simulink model "ProgettoCompleto"  (R2022b)
settings: Solver=ode1  StartTime=0.0  StopTime=inf  FixedStep=0.001  RelTol=1e-9
PreLoadFcn:
  | params
InitFcn:
  | params
model workspace (MAT data in the model file):
  SL_ROS_VariableLengthArrays_MaxSizes.CommonInfo.ArrayTruncateAction = 'EmitWarning'
  SL_ROS_VariableLengthArrays_MaxSizes.MsgTypeMap = containers.Map
  SL_ROS_VariableLengthArrays_MaxSizes.MsgTypeMap.serialization.keys = {'sensor_msgs/CompressedImage'}
  SL_ROS_VariableLengthArrays_MaxSizes.MsgTypeMap.serialization.values{1}(1).PropertyName = 'Data'
  SL_ROS_VariableLengthArrays_MaxSizes.MsgTypeMap.serialization.values{1}(1).DataType = 'uint8'
  SL_ROS_VariableLengthArrays_MaxSizes.MsgTypeMap.serialization.values{1}(1).MaxLength = 300000
  SL_ROS_VariableLengthArrays_MaxSizes.MsgTypeMap.serialization.values{1}(2).PropertyName = 'Format'
  SL_ROS_VariableLengthArrays_MaxSizes.MsgTypeMap.serialization.values{1}(2).DataType = 'uint8'
  SL_ROS_VariableLengthArrays_MaxSizes.MsgTypeMap.serialization.values{1}(2).MaxLength = 128
  SL_ROS_VariableLengthArrays_MaxSizes.MsgTypeMap.serialization.uniformity = 0
  SL_ROS_VariableLengthArrays_MaxSizes.MsgTypeMap.serialization.keyType = 'char'
  SL_ROS_VariableLengthArrays_MaxSizes.MsgTypeMap.serialization.valueType = 'any'
undefined symbols (not defined in the file): gray, L, r, Rec, SDTV, sigbuilder_block, VelLeft, VelRight
libraries: robotlib x8, simulink_extras x8, dspstat3 x4, visiontextngfix x3, slpidlib x3, visiontransforms x2, visionconversions x2, dspmtrx3 x2, visionfilter x1, matrix_library x1, visionanalysis x1, visionstatistics x1
settings Model: Creator=domen  LastModifiedBy=gaetano
settings OptimizationCC: EnhancedBackFolding=on  PassReuseOutputArgsAs=Individual arguments  ZeroExternalMemoryAtStartup=off  ZeroInternalMemoryAtStartup=off  MaxStackSize=64  OptimizeBlockOrder=speed  DifferentSizesBufferReuse=on  OptimizationCustomize=off  EfficientTunableParamExpr=on
settings DebuggingCC: ParameterTunabilityLossMsg=error
settings HardwareCC: ProdBitPerPointer=32  ProdBitPerSizeT=32  ProdBitPerPtrDiffT=32  ProdLargestAtomicFloat=None  ProdIntDivRoundTo=Undefined  ProdEndianess=Unspecified  ProdWordSize=32  ProdHWDeviceType=Generic->Unspecified (assume 32-bit Generic)  UseEmbeddedCoderFeatures=off
settings RTWCC: Description=Embedded Coder  SystemTargetFile=ert.tlc  HardwareBoard=Robot Operating System (ROS)  TLCOptions="-aInlineSetEventsForThisBaseRateFcn=TLC_FALSE -aSuppressMultiTaskScheduler=TLC_FALSE  -aRateBasedStepFcn=0"  TemplateMakefile=ert_default_tmf  Toolchain=Catkin  TargetLang=C++
settings CodeAppCC: ForceParamTrailComments=on  IgnoreCustomStorageClasses=off  OperatorAnnotations=on  SimulinkDataObjDesc=on  SFDataObjDesc=on  InsertBlockDesc=on
settings ERTTargetCC: SupportNonInlinedSFcns=on

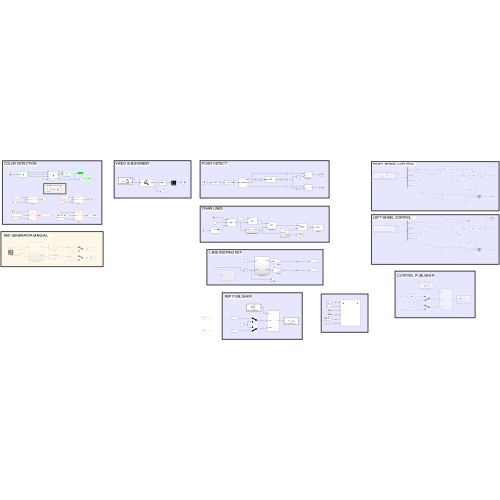
[thumbnail: Simulink's stored preview of the top-level diagram]
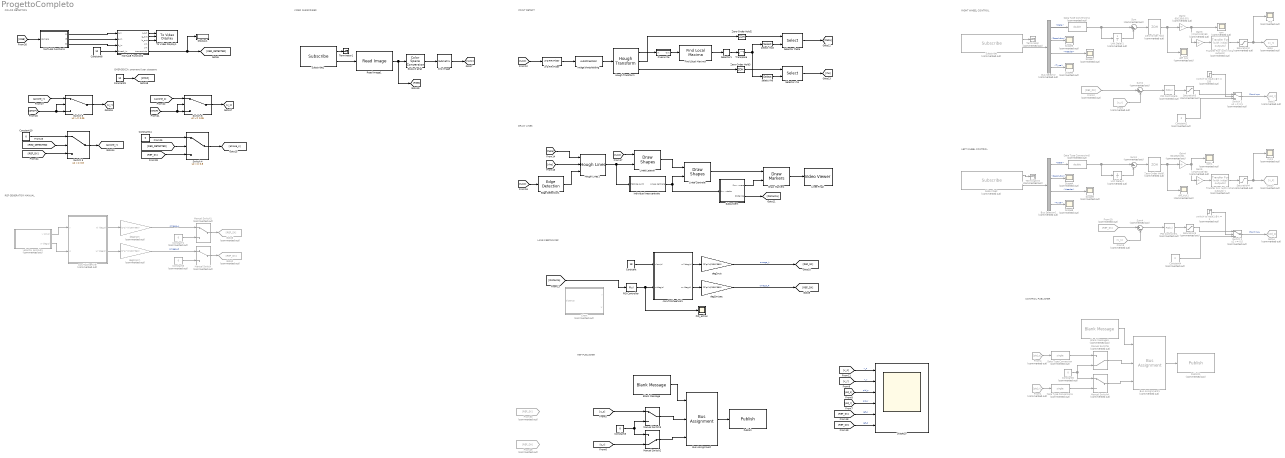
== system ProgettoCompleto ==
  note: VIDEO SUBSCRIBER
  note: POINT DETECT
  note: DRAW LINES
  note: LANE KEEPING REF
  note: REF PUBLISHER
  note: CONTROL PUBLISHER
  note: EMERGENZA: premere 0 per stoppare
  note: COLOR DETECTION
  note: REF GENERATOR MANUAL
  note: RIGHT WHEEL CONTROL
  note: LEFT WHEEL CONTROL
  2-D FIR Filter : visionfilter/2-D FIR Filter  separable=off  filtSrc=Specify via dialog  filterMtrx=[-1 0 1]  verticalFilter=[4 0]  horizontalFilter=[4 0]  outSize=Same as input port I  padType=Replicate  padSrc=Specify via dialog  padVal=0  method=Convolution  firstCoeffMode=Specify word length  firstCoeffWordLength=16  firstCoeffFracLength=14  firstCoeffSignedness=Signed  firstCoeffLastDataTypeStr=fixdt(1,16)  outputSignedness=Auto  accumLastDataTypeStr=Inherit: Same as product output  prodOutputMode=Binary point scaling  prodOutputWordLength=32  prodOutputFracLength=10  prodOutputLastDataTypeStr=fixdt([],32,10)  roundingMode=Floor  overflowMode=on  firstCoeffDataTypeStr=fixdt(1,16)  firstCoeffMin=[]  firstCoeffMax=[]  prodOutputDataTypeStr=fixdt([],32,10)  accumDataTypeStr=Inherit: Same as product output  outputMin=[]  outputMax=[]
  Blank Message : robotlib/Blank Message  messageClass=Message  entityType=duckietown_msgs/WheelsCmdStamped  messageType=duckietown_msgs/WheelsCmdStamped  SampleTime=-1  legacyBusStruct=off
      settings: LibrarySourceBlock=roslib/ROS/Blank Message
  Blank Message1 : robotlib/Blank Message  Commented=on  messageClass=Message  entityType=duckietown_msgs/WheelsCmdStamped  messageType=duckietown_msgs/WheelsCmdStamped  SampleTime=-1  legacyBusStruct=off
      settings: LibrarySourceBlock=roslib/ROS/Blank Message
  Bus Assignment : BusAssignment  AssignedSignals=VelLeft,VelRight
  Bus Assignment1 : BusAssignment  Commented=on  AssignedSignals=VelLeft,VelRight
  Bus Selector : BusSelector  Commented=on  OutputSignals=Data,Resolution,Header,Type
  Bus Selector1 : BusSelector  Commented=on  OutputSignals=Data,Resolution,Header,Type
  Chart : Stateflow chart  Commented=on  TreatAsAtomicUnit=on
  Clip image : matrix_library/Submatrix  RowSpan=Range of rows  RowStartMode=Offset from middle  RowStartIndex=15  RowEndMode=Last  RowEndIndex=1  ColSpan=All columns  ColStartMode=First  ColStartIndex=1  ColEndMode=Last  ColEndIndex=1
  Constant : Constant  Value=18
  Constant{1..2,4..5} (4 alike) : Constant  Commented=on  Value=0
  Constant10 : Constant  Value=0
  Constant11 : Constant  Value=0
  Constant3 : Constant  Value=0  OutDataTypeStr=single
  Constant6 : Constant  Commented=on  Value=0  OutDataTypeStr=single
  Constant8 : Constant  Value=10
  Constant9 : Constant  Value=10
  Data Type Conversion : DataTypeConversion  Commented=on  OutDataTypeStr=single  SaturateOnIntegerOverflow=off  RndMeth=Floor
  Data Type Conversion1 : DataTypeConversion  Commented=on  OutDataTypeStr=single  SaturateOnIntegerOverflow=off  RndMeth=Floor
  Data Type Conversion4 : DataTypeConversion  Commented=on  OutDataTypeStr=double  SaturateOnIntegerOverflow=off  RndMeth=Floor
  Data Type Conversion5 : DataTypeConversion  Commented=on  OutDataTypeStr=double  SaturateOnIntegerOverflow=off  RndMeth=Floor
  Display1 : Display
  Draw Markers : visiontextngfix/Draw Markers  shape=X-mark  size=3  fill=off  fillClrSource=Specify via dialog  display=White  intensity=200  color=[250 0 0]  opacity=0.6  viewport=Entire image  antialiasing=off  inType=Obsolete  imagePorts=One multidimensional signal  roundingMode=Floor  overflowMode=off  memoryMode=Specify word length  memoryWordLength=16  memoryFracLength=15  prodOutputMode=Binary point scaling  prodOutputWordLength=32  prodOutputFracLength=14
  Edge Detection1 : visionanalysis/Edge Detection  method=Sobel  outputType=Binary image  userDefinedThreshold=off  thresholdSource=Input port  threshold=20  thresholdTuning=4  edgeThinning=off  threshold_canny=[0.25 0.60]  autoPercent=70  sigma=1  roundingMode=Floor  overflowMode=off  prodOutputMode=Binary point scaling  prodOutputWordLength=32  prodOutputFracLength=8
  Find Local Maxima : visionstatistics/Find Local Maxima  num_peaks=2  nhood_size=[301 81]  src_thresh=Obsolete9b  src_thresh_inuse=Specify via dialog  threshold=1  inputIsHough=on  dt_peak=uint16  isOutVarDim=on  dt_count=uint16
  From : From  Commented=on  GotoTag=v_r
  From1 : From  Commented=on  GotoTag=pid_r
  From10 : From  Commented=on  GotoTag=REF_SX
  From2 : From  Commented=on  GotoTag=REF_DX
  From29 : From  Commented=on  GotoTag=REF_DX
  From3 : From  Commented=on  GotoTag=v_s
  From30 : From  Commented=on  GotoTag=REF_SX
  From4 : From  Commented=on  GotoTag=pid_s
  Gain2 : Gain  Commented=on  Gain=60/135/0.001
  Gain3 : Gain  Commented=on  Gain=(2*pi*0.03)/60
  Gain4 : Gain  Commented=on  Gain=60/135/0.001
  Gain5 : Gain  Commented=on  Gain=(2*pi*0.03)/60
  Goto : Goto  Commented=on  GotoTag=v_r
  Goto1 : Goto  Commented=on  GotoTag=pid_r
  Goto2 : Goto  Commented=on  GotoTag=REF_DX
  Goto3 : Goto  Commented=on  GotoTag=v_s
  Goto4 : Goto  Commented=on  GotoTag=pid_s
  Goto6 : Goto  Commented=on  GotoTag=REF_SX
  Hough Lines1 : visiontransforms/Hough Lines  sineCompMethod=Trigonometric function  thetaRes=pi/180  roundingMode=Nearest  overflowMode=on  firstCoeffMode=Specify word length  firstCoeffWordLength=16  prodOutputMode=Binary point scaling  prodOutputWordLength=32  prodOutputFracLength=16  firstCoeffFracLength=15
  Hough Transform : visiontransforms/Hough Transform  theta_res=pi/180  rho_res=1  out_theta_rho=on  outdtmode=single  roundingMode=Nearest  overflowMode=on  firstCoeffMode=Binary point scaling  firstCoeffWordLength=16  firstCoeffFracLength=14  secondCoeffMode=Binary point scaling  secondCoeffWordLength=32  secondCoeffFracLength=16  prodOutputMode=Binary point scaling  prodOutputWordLength=32  prodOutputFracLength=20  accumMode=Binary point scaling  accumWordLength=32  accumFracLength=20  outputMode=Binary point scaling  outputWordLength=16  outputFracLength=0  memoryMode=Binary point scaling  memoryWordLength=32  memoryFracLength=16
  Image thresholding : visionconversions/Autothreshold  operator=>  threshOut=off  effMetricOut=off  userDefinedRange=off  umin=50  umax=255  outOfRngOpt=Ignore  scaleThreshold=off  scaleFactor=1  roundingMode=Floor  overflowMode=off  P1Mode=Specify word length  P1WordLength=32  P1FracLength=30  P2Mode=Specify word length  P2WordLength=32  P2FracLength=22  P3Mode=Specify word length  P3WordLength=32  P3FracLength=14  P4Mode=Binary point scaling  P4WordLength=32  P4FracLength=15  Q1Mode=Specify word length  Q1WordLength=32  Q1FracLength=16  EMMode=Specify word length  EMWordLength=16  EMFracLength=14
  Individua linea centrale : Subsystem
  Linea Centrale : visiontextngfix/Draw Shapes  shape=Lines  fill=off  lineWidth=2  fillClrSource=Specify via dialog  display=White  intensity=200  color=[200 255 100]  opacity=0.6  viewport=Entire image  antialiasing=off  inType=Obsolete  imagePorts=One multidimensional signal  roundingMode=Floor  overflowMode=off  memoryMode=Specify word length  memoryWordLength=16  prodOutputMode=Binary point scaling  prodOutputWordLength=32  prodOutputFracLength=14  memoryFracLength=15
  Linee Finali : VideoViewer  colormapValue=gray(256)  FigPos=[342 823 793 695]
  Linee Laterali : visiontextngfix/Draw Shapes  shape=Lines  fill=off  lineWidth=2  fillClrSource=Specify via dialog  display=White  intensity=200  color=[200 255 100]  opacity=0.6  viewport=Entire image  antialiasing=off  inType=Obsolete  imagePorts=One multidimensional signal  roundingMode=Floor  overflowMode=off  memoryMode=Specify word length  memoryWordLength=16  prodOutputMode=Binary point scaling  prodOutputWordLength=32  prodOutputFracLength=14  memoryFracLength=15
  MATLAB Function1 : MATLAB Function  TreatAsAtomicUnit=on
  MATLAB Function2 : MATLAB Function  TreatAsAtomicUnit=on
  Manual Switch : ManualSwitch  Commented=on
  Manual Switch1 : ManualSwitch  Commented=on
  Manual Switch2 : ManualSwitch  CurrentSetting=0
  Manual Switch3 : ManualSwitch
  Manual Switch4 : ManualSwitch  Commented=on
  Manual Switch5 : ManualSwitch  Commented=on  CurrentSetting=0
  Overwrite : Subsystem
  PID Controller : slpidlib/PID Controller  Controller=P  Form=Parallel  TimeDomain=Continuous-time  UseExternalTs=off  SampleTime=-1  IntegratorMethod=Forward Euler  FilterMethod=Forward Euler  ControllerParametersSource=internal  P=0.70  I=1  UseKiTs=off  D=0.10  N=100  UseFilter=on  TunerSelectOption=Transfer Function Based (PID Tuner App)  InitialConditionSource=internal  InitialConditionForIntegrator=0  InitialConditionForFilter=0  DifferentiatorICPrevScaledInput=0  ExternalReset=none  TrackingMode=off  Kt=1  LimitOutput=off  SatLimitsSource=internal  UpperSaturationLimit=40  LowerSaturationLimit=-40  LinearizeAsGain=off  AntiWindupMode=none  Kb=1  LimitIntegrator=off  UpperIntegratorSaturationLimit=inf  LowerIntegratorSaturationLimit=-inf  PGainOutDataTypeStr=double  PProdOutDataTypeStr=double  POutMin=[]  POutMax=[]  IOutMin=[]  IOutMax=[]  DOutMin=[]  DOutMax=[]  NOutMin=[]  NOutMax=[]  SumOutMin=[]  SumOutMax=[]  SaturationOutMin=[]  SaturationOutMax=[]  PParamMin=[]  PParamMax=[]  IParamMin=[]  IParamMax=[]  DParamMin=[]  DParamMax=[]  NParamMin=[]  NParamMax=[]  KbParamMin=[]  KbParamMax=[]  KtParamMin=[]  KtParamMax=[]  KbOutMin=[]  KbOutMax=[]  KtOutMin=[]  KtOutMax=[]  IntegratorOutMin=[]  IntegratorOutMax=[]  FilterOutMin=[]  FilterOutMax=[]  SumI1OutMin=[]  SumI1OutMax=[]  SumI2OutMin=[]  SumI2OutMax=[]  SumI3OutMin=[]  SumI3OutMax=[]  SumI4OutMin=[]  SumI4OutMax=[]  SumDOutMin=[]  SumDOutMax=[]  DifferentiatorOutMin=[]  DifferentiatorOutMax=[]  FilterDiffOutCoefMin=[]  FilterDiffOutCoefMax=[]  ReciprocalOutMin=[]  ReciprocalOutMax=[]  SumDenOutMin=[]  SumDenOutMax=[]  SumNumOutMin=[]  SumNumOutMax=[]  DivideOutMin=[]  DivideOutMax=[]  UdiffTsProdOutMin=[]  UdiffTsProdOutMax=[]  NTsProdOutMin=[]  NTsProdOutMax=[]  UintegralTsProdOutMin=[]  UintegralTsProdOutMax=[]  UngainTsProdOutMin=[]  UngainTsProdOutMax=[]  ClampingZeroOutDataTypeStr=Inherit: Inherit via back propagation  ClampingZeroOutMin=[]  ClampingZeroOutMax=[]  FilterDenConstantOutDataTypeStr=Inherit: Inherit via back propagation  FilterDenConstantOutMin=[]  FilterDenConstantOutMax=[]  PCopyOutDataTypeStr=Inherit: Inherit via back propagation  PCopyOutMin=[]  PCopyOutMax=[]  NCopyOutDataTypeStr=Inherit: Inherit via back propagation  NCopyOutMin=[]  NCopyOutMax=[]  IntegratorContinuousStateAttributes=''  IntegratorStateMustResolveToSignalObject=off  IntegratorRTWStateStorageClass=Auto  FilterContinuousStateAttributes=''  FilterStateMustResolveToSignalObject=off  FilterRTWStateStorageClass=Auto  ParallelPVariant=InternalParameters  IdealPVariant=Disabled  IVariant=Disabled  DVariant=Disabled  IntegratorVariant=Disabled  SatVariant=Disabled  AWVariant=Disabled  PCopyVariant=Disabled  TRVariant=Disabled  FdbkBlocksVariant=Forward  IdealPFdbkVariant=Disabled  SatFdbkVariant=Disabled  DerivativeFilterVariant=Disabled  NVariant=Disabled  NCopyVariant=Disabled_SignalSpec  FilterICVariant=Disabled  IntegratorICVariant=Disabled  ExternalResetVariant=Disabled  TRSumVariant=Passthrough  SumFdbkVariant=Disabled  SumVariant=Passthrough_P  TsampFilterVariant=InternalTs  TsampNgainVariant=Passthrough  TsampIntegralVariant=Disabled_SignalSpec  ExternalSaturationOutDataTypeStr=Inherit: Same as second input
  PID Controller1 : slpidlib/PID Controller  Commented=on  Controller=PID  Form=Parallel  TimeDomain=Continuous-time  UseExternalTs=off  SampleTime=-1  IntegratorMethod=Forward Euler  FilterMethod=Forward Euler  ControllerParametersSource=internal  P=1.9500021729767  I=2.64652436503106  UseKiTs=off  D=0.143645278367384  N=3.78681783159113  UseFilter=on  TunerSelectOption=Transfer Function Based (PID Tuner App)  InitialConditionSource=internal  InitialConditionForIntegrator=0  InitialConditionForFilter=0  DifferentiatorICPrevScaledInput=0  ExternalReset=none  TrackingMode=off  Kt=1  LimitOutput=off  SatLimitsSource=internal  UpperSaturationLimit=inf  LowerSaturationLimit=-inf  LinearizeAsGain=on  AntiWindupMode=none  Kb=1  LimitIntegrator=off  UpperIntegratorSaturationLimit=inf  LowerIntegratorSaturationLimit=-inf  POutMin=[]  POutMax=[]  IOutMin=[]  IOutMax=[]  DOutMin=[]  DOutMax=[]  NOutMin=[]  NOutMax=[]  SumOutMin=[]  SumOutMax=[]  SaturationOutMin=[]  SaturationOutMax=[]  PParamMin=[]  PParamMax=[]  IParamMin=[]  IParamMax=[]  DParamMin=[]  DParamMax=[]  NParamMin=[]  NParamMax=[]  KbParamMin=[]  KbParamMax=[]  KtParamMin=[]  KtParamMax=[]  KbOutMin=[]  KbOutMax=[]  KtOutMin=[]  KtOutMax=[]  IntegratorOutMin=[]  IntegratorOutMax=[]  FilterOutMin=[]  FilterOutMax=[]  SumI1OutMin=[]  SumI1OutMax=[]  SumI2OutMin=[]  SumI2OutMax=[]  SumI3OutMin=[]  SumI3OutMax=[]  SumI4OutMin=[]  SumI4OutMax=[]  SumDOutMin=[]  SumDOutMax=[]  DifferentiatorOutMin=[]  DifferentiatorOutMax=[]  FilterDiffOutCoefMin=[]  FilterDiffOutCoefMax=[]  ReciprocalOutMin=[]  ReciprocalOutMax=[]  SumDenOutMin=[]  SumDenOutMax=[]  SumNumOutMin=[]  SumNumOutMax=[]  DivideOutMin=[]  DivideOutMax=[]  UdiffTsProdOutMin=[]  UdiffTsProdOutMax=[]  NTsProdOutMin=[]  NTsProdOutMax=[]  UintegralTsProdOutMin=[]  UintegralTsProdOutMax=[]  UngainTsProdOutMin=[]  UngainTsProdOutMax=[]  ClampingZeroOutDataTypeStr=Inherit: Inherit via back propagation  ClampingZeroOutMin=[]  ClampingZeroOutMax=[]  FilterDenConstantOutDataTypeStr=Inherit: Inherit via back propagation  FilterDenConstantOutMin=[]  FilterDenConstantOutMax=[]  PCopyOutDataTypeStr=Inherit: Inherit via back propagation  PCopyOutMin=[]  PCopyOutMax=[]  NCopyOutDataTypeStr=Inherit: Inherit via back propagation  NCopyOutMin=[]  NCopyOutMax=[]  IntegratorContinuousStateAttributes=''  IntegratorStateMustResolveToSignalObject=off  IntegratorRTWStateStorageClass=Auto  FilterContinuousStateAttributes=''  FilterStateMustResolveToSignalObject=off  FilterRTWStateStorageClass=Auto  ParallelPVariant=InternalParameters  IdealPVariant=Disabled  IVariant=InternalParameters  DVariant=InternalParameters  IntegratorVariant=Continuous  SatVariant=Disabled  AWVariant=Passthrough  PCopyVariant=Disabled  TRVariant=Disabled  FdbkBlocksVariant=Forward  IdealPFdbkVariant=Disabled  SatFdbkVariant=Disabled  DerivativeFilterVariant=ContFilter  NVariant=InternalParameters  NCopyVariant=Disabled  FilterICVariant=InternalICsFilter  IntegratorICVariant=InternalICs  ExternalResetVariant=Disabled  TRSumVariant=Passthrough  SumFdbkVariant=Disabled  SumVariant=Sum_PID  TsampFilterVariant=InternalTs  TsampNgainVariant=Passthrough  TsampIntegralVariant=Passthrough  ExternalSaturationOutDataTypeStr=Inherit: Same as second input
  PID Controller5 : slpidlib/PID Controller  Commented=on  Controller=PID  Form=Parallel  TimeDomain=Continuous-time  UseExternalTs=off  SampleTime=-1  IntegratorMethod=Forward Euler  FilterMethod=Forward Euler  ControllerParametersSource=internal  P=1.9500021729767  I=2.64652436503106  UseKiTs=off  D=0.143645278367384  N=3.78681783159113  UseFilter=on  TunerSelectOption=Transfer Function Based (PID Tuner App)  InitialConditionSource=internal  InitialConditionForIntegrator=0  InitialConditionForFilter=0  DifferentiatorICPrevScaledInput=0  ExternalReset=none  TrackingMode=off  Kt=1  LimitOutput=off  SatLimitsSource=internal  UpperSaturationLimit=inf  LowerSaturationLimit=-inf  LinearizeAsGain=on  AntiWindupMode=none  Kb=1  LimitIntegrator=off  UpperIntegratorSaturationLimit=inf  LowerIntegratorSaturationLimit=-inf  POutMin=[]  POutMax=[]  IOutMin=[]  IOutMax=[]  DOutMin=[]  DOutMax=[]  NOutMin=[]  NOutMax=[]  SumOutMin=[]  SumOutMax=[]  SaturationOutMin=[]  SaturationOutMax=[]  PParamMin=[]  PParamMax=[]  IParamMin=[]  IParamMax=[]  DParamMin=[]  DParamMax=[]  NParamMin=[]  NParamMax=[]  KbParamMin=[]  KbParamMax=[]  KtParamMin=[]  KtParamMax=[]  KbOutMin=[]  KbOutMax=[]  KtOutMin=[]  KtOutMax=[]  IntegratorOutMin=[]  IntegratorOutMax=[]  FilterOutMin=[]  FilterOutMax=[]  SumI1OutMin=[]  SumI1OutMax=[]  SumI2OutMin=[]  SumI2OutMax=[]  SumI3OutMin=[]  SumI3OutMax=[]  SumI4OutMin=[]  SumI4OutMax=[]  SumDOutMin=[]  SumDOutMax=[]  DifferentiatorOutMin=[]  DifferentiatorOutMax=[]  FilterDiffOutCoefMin=[]  FilterDiffOutCoefMax=[]  ReciprocalOutMin=[]  ReciprocalOutMax=[]  SumDenOutMin=[]  SumDenOutMax=[]  SumNumOutMin=[]  SumNumOutMax=[]  DivideOutMin=[]  DivideOutMax=[]  UdiffTsProdOutMin=[]  UdiffTsProdOutMax=[]  NTsProdOutMin=[]  NTsProdOutMax=[]  UintegralTsProdOutMin=[]  UintegralTsProdOutMax=[]  UngainTsProdOutMin=[]  UngainTsProdOutMax=[]  ClampingZeroOutDataTypeStr=Inherit: Inherit via back propagation  ClampingZeroOutMin=[]  ClampingZeroOutMax=[]  FilterDenConstantOutDataTypeStr=Inherit: Inherit via back propagation  FilterDenConstantOutMin=[]  FilterDenConstantOutMax=[]  PCopyOutDataTypeStr=Inherit: Inherit via back propagation  PCopyOutMin=[]  PCopyOutMax=[]  NCopyOutDataTypeStr=Inherit: Inherit via back propagation  NCopyOutMin=[]  NCopyOutMax=[]  IntegratorContinuousStateAttributes=''  IntegratorStateMustResolveToSignalObject=off  IntegratorRTWStateStorageClass=Auto  FilterContinuousStateAttributes=''  FilterStateMustResolveToSignalObject=off  FilterRTWStateStorageClass=Auto  ParallelPVariant=InternalParameters  IdealPVariant=Disabled  IVariant=InternalParameters  DVariant=InternalParameters  IntegratorVariant=Continuous  SatVariant=Disabled  AWVariant=Passthrough  PCopyVariant=Disabled  TRVariant=Disabled  FdbkBlocksVariant=Forward  IdealPFdbkVariant=Disabled  SatFdbkVariant=Disabled  DerivativeFilterVariant=ContFilter  NVariant=InternalParameters  NCopyVariant=Disabled  FilterICVariant=InternalICsFilter  IntegratorICVariant=InternalICs  ExternalResetVariant=Disabled  TRSumVariant=Passthrough  SumFdbkVariant=Disabled  SumVariant=Sum_PID  TsampFilterVariant=InternalTs  TsampNgainVariant=Passthrough  TsampIntegralVariant=Passthrough  ExternalSaturationOutDataTypeStr=Inherit: Same as second input
  PID_action : Scope
  Publish : robotlib/Publish  topicSource=Select from ROS network  topic=/vic9osimhen/wheels_driver_node/wheels_cmd  messageType=duckietown_msgs/WheelsCmdStamped  legacyBusStruct=off  messageQueueLength=1
      settings: LibrarySourceBlock=roslib/ROS/Publish
  Publish1 : robotlib/Publish  Commented=on  topicSource=Select from ROS network  topic=/vic9osimhen/wheels_driver_node/wheels_cmd  messageType=duckietown_msgs/WheelsCmdStamped  legacyBusStruct=off  messageQueueLength=1
      settings: LibrarySourceBlock=roslib/ROS/Publish
  Read Image1 : robotlib/Read Image  MaximumImageSize=[480,640]  ImageEncoding=rgb8  ShowAlphaOutput=off  ShowErrorCodeOutput=off  VariableSizeOutputs=off
      settings: LibrarySourceBlock=roslib/ROS/Read Image
  Saturation{2..5} (4 alike) : Saturate  Commented=on  UpperLimit=0.95  LowerLimit=-0.95
  Scala di grigi : visionconversions/Color Space  Conversion  conversion=Obsolete  conversionActive=R'G'B' to intensity  wp_str=D65  rec=Rec. 601 (SDTV)  sys=1125/60/2:1  imagePorts=One multidimensional signal
  Scope10 : Scope  NumInputPorts=6
  Scope{4..9} (6 alike) : Scope  Commented=on
  Selector rho : Selector  NumberOfDimensions=2  InputPortWidth=3  IndexOptions=Select all,Index vector (port)  Indices=1,2  OutputSizes=1,1
  Selector theta : Selector  NumberOfDimensions=2  InputPortWidth=3  IndexOptions=Select all,Index vector (port)  Indices=1,2  OutputSizes=1,1
  Selector1 : Selector  NumberOfDimensions=2  InputPortWidth=3  IndexOptions=Select all,Index vector (dialog)  Indices=[2 1],[2 1]  OutputSizes=1,1
  Subscribe : robotlib/Subscribe  Commented=on  topicSource=Select from ROS network  topic=/vic9osimhen/right_wheel_encoder_node/tick  messageType=duckietown_msgs/WheelEncoderStamped  SampleTime=-1  legacyBusStruct=off  messageQueueLength=1
      settings: LibrarySourceBlock=roslib/ROS/Subscribe
  Subscribe1 : robotlib/Subscribe  topicSource=Select from ROS network  topic=/vic9osimhen/camera_node/image/compressed  messageType=sensor_msgs/CompressedImage  SampleTime=-1  legacyBusStruct=off  messageQueueLength=1
      settings: LibrarySourceBlock=roslib/ROS/Subscribe
  Subscribe2 : robotlib/Subscribe  Commented=on  topicSource=Select from ROS network  topic=/vic9osimhen/left_wheel_encoder_node/tick  messageType=duckietown_msgs/WheelEncoderStamped  SampleTime=-1  legacyBusStruct=off  messageQueueLength=1
      settings: LibrarySourceBlock=roslib/ROS/Subscribe
  Subsystem : Subsystem
  Sum{,2..4} (4 alike) : Sum  Commented=on  Inputs=|+-
  Switch 1 : Switch  Commented=on  Threshold=0.5  SaturateOnIntegerOverflow=off  InputSameDT=off
  Switch 2 : Switch  Commented=on  Threshold=0.5  SaturateOnIntegerOverflow=off  InputSameDT=off
  Switch 3 : Switch  Threshold=0.8  SaturateOnIntegerOverflow=off  InputSameDT=off
  Switch 4 : Switch  Threshold=0.8  SaturateOnIntegerOverflow=off  InputSameDT=off
  Switch 5 : Switch  Threshold=0.05  SaturateOnIntegerOverflow=off  InputSameDT=off
  Switch 6 : Switch  Threshold=0.05  SaturateOnIntegerOverflow=off  InputSameDT=off
  Terminator : Terminator  Commented=on
  Terminator1 : Terminator
  Terminator3 : Terminator  Commented=on
  To Video Display1 : visionsinks/To Video Display  windowSizeMode=Normal  openAtMdlStart=on  fullScreen=off  videoWindowX=1186  videoWindowY=599  saveWindowSize=off  videoWindowWidth=640  videoWindowHeight=480  inputColorFormat=RGB  inputType=Obsolete  imagePorts=Separate color signals  OutputDevice=On-screen video monitor  dataOrg=Column-major  isWindowOpen=off
  Transfer Fcn (with initial outputs) : simulink_extras/Additional Linear/Transfer Fcn (with initial outputs)  Commented=on  N=[1]  D="[1  1]"  Y0=0  U0=0
  Transfer Fcn (with initial outputs)1 : simulink_extras/Additional Linear/Transfer Fcn (with initial outputs)  Commented=on  N=[1]  D="[1  1]"  Y0=0  U0=0
  Transpose : Math  Operator=transpose  SignedPower=on
  Unit Delay1 : UnitDelay  Commented=on  SampleTime=-1  HasFrameUpgradeWarning=on
  Unit Delay2 : UnitDelay  Commented=on  SampleTime=-1  HasFrameUpgradeWarning=on
  Zero-Order Hold : ZeroOrderHold  Commented=on  SampleTime=-1
  Zero-Order Hold1 : ZeroOrderHold  Commented=on  SampleTime=-1
  Zero-Order Hold2 : ZeroOrderHold  SampleTime=-1
  Zero-Order Hold3 : ZeroOrderHold  SampleTime=-1
  convToWheelVel : Subsystem  Commented=on
  convToWheelVel1 : Subsystem
  deg2m/s : Gain  Gain=(2*pi*r)/(100*360)
  deg2m/sec : Gain  Gain=(2*pi*r)/(100*360)
  deg2rpm : Gain  Commented=on  Gain=(2*pi*r)/(100*360)
  deg2rpm1 : Gain  Commented=on  Gain=(2*pi*r)/(100*360)
  diff_tick : Scope  Commented=on
  diff_tick1 : Scope  Commented=on
  m/s : Scope  Commented=on
  m/s1 : Scope  Commented=on
  rpm : Scope  Commented=on
  rpm1 : Scope  Commented=on
  select rho : Selector  NumberOfDimensions=2  InputPortWidth=3  IndexOptions=Index vector (dialog),Select all  Indices=1,-1  OutputSizes=1
  select rho3 : Selector  NumberOfDimensions=2  InputPortWidth=3  IndexOptions=Index vector (dialog),Select all  Indices=2,-1  OutputSizes=1
  switch to input1 @ t = 1 : Step  Commented=on  Time=15  SampleTime=0
  switch to input1 @ t = 150 : Step  Commented=on  Time=15  SampleTime=0
  velocita_assoluta : Subsystem  Tag=STV Subsys  Commented=on  LoadFcn=sigbuilder_block('load');  StartFcn=sigbuilder_block('start');  StopFcn=sigbuilder_block('stop');  ClipboardFcn=sigbuilder_block('clipboard');  mask(Sigbuilder block){tuvar=[0:10]}
      mask help: Simulink:masks:SigbuilderBlock_MD
      mask init:
      | if ~strcmp(get_param(bdroot(gcbh),'SimulationStatus'),'stopped') tuvar = sigbuilder_block('maskInit'); end
      settings: CopyFcn=sigbuilder_block('copy');  DeleteFcn=sigbuilder_block('delete');  ModelCloseFcn=sigbuilder_block('modelClose');  PreSaveFcn=sigbuilder_block('preSave');  PauseFcn=sigbuilder_block('pause');  ContinueFcn=sigbuilder_block('continue');  NameChangeFcn=sigbuilder_block('namechange');  OpenFcn=sigbuilder_block('open',[0 72 1440 724 ]);  CloseFcn=sigbuilder_block('close');
      mask Display: plot(0, 0, 100, 100,[2, 2, 32, 32, 2], [68, 8, 8, 68, 68],[32, 2], [38, 38], [32, 19, 2],[53, 60, 44], [32, 17, 17, 2],[16, 16, 31, 31]);txt = getActiveGroup(gcbh);text(2, 100, txt,'verticalAlignment', 'top');
  wires:
  Bus Assignment/1 -> Publish/1
  Blank Message/1 -> Bus Assignment/1
  Subscribe/1 -> Terminator/1
  Subscribe/2 -> Bus Selector/1
  Bus Selector/2 -> Scope5/1  "<Resolution>"
  Bus Selector/3 -> Scope7/1  "<Header>"
  Bus Selector/4 -> Scope6/1  "<Type>"
  Bus Selector/1 -> Data Type Conversion4/1  "<Data>"
  Sum/1 -> Zero-Order Hold/1
  Gain2/1 -> Gain3/1, rpm/1
  Gain3/1 -> Transfer Fcn (with initial outputs)/1
  Zero-Order Hold/1 -> Gain2/1, diff_tick/1
  Transfer Fcn (with initial outputs)/1 -> Saturation2/1
  Unit Delay1/1 -> Sum/2
  Data Type Conversion4/1 -> Unit Delay1/1, Sum/1
  Constant2/1 -> Switch 1/3
  switch to input1 @ t = 150/1 -> Switch 1/2
  Switch 1/1 -> Goto1/1  "Plant inpu"
  Saturation2/1 -> m/s/1, Goto/1
  From/1 -> Sum2/2
  Sum2/1 -> PID Controller5/1
  PID Controller5/1 -> Saturation3/1
  Saturation3/1 -> Switch 1/1
  Subscribe2/1 -> Terminator3/1
  Bus Selector1/1 -> Data Type Conversion5/1  "<Data>"
  Bus Selector1/4 -> Scope8/1  "<Type>"
  Subscribe2/2 -> Bus Selector1/1
  Gain5/1 -> Transfer Fcn (with initial outputs)1/1
  Bus Selector1/3 -> Scope9/1  "<Header>"
  Zero-Order Hold1/1 -> Gain4/1, diff_tick1/1
  Gain4/1 -> Gain5/1, rpm1/1
  Unit Delay2/1 -> Sum3/2
  Transfer Fcn (with initial outputs)1/1 -> Saturation4/1
  Data Type Conversion5/1 -> Unit Delay2/1, Sum3/1
  switch to input1 @ t = 1/1 -> Switch 2/2
  Bus Selector1/2 -> Scope4/1  "<Resolution>"
  Saturation4/1 -> m/s1/1, Goto3/1
  Switch 2/1 -> Goto4/1  "Plant inpu"
  Sum3/1 -> Zero-Order Hold1/1
  Constant4/1 -> Switch 2/3
  Sum4/1 -> PID Controller1/1
  From3/1 -> Sum4/2
  PID Controller1/1 -> Saturation5/1
  Saturation5/1 -> Switch 2/1
  Constant5/1 -> Manual Switch/2
  velocita_assoluta/1(v (cm/s)) -> convToWheelVel/1(v)
  convToWheelVel/1(wl (deg/s)) -> deg2rpm/1
  convToWheelVel/2(wr (deg/s)) -> deg2rpm1/1
  Constant1/1 -> Manual Switch1/2
  Manual Switch1/1 -> Goto6/1
  Manual Switch/1 -> Goto2/1
  deg2rpm/1 -> Manual Switch1/1  "omega_L"
  deg2rpm1/1 -> Manual Switch/1  "omega_R"
  velocita_assoluta/2(w (deg/s)) -> convToWheelVel/2(w)
  Constant3/1 -> Manual Switch2/1, Manual Switch3/2
  Subscribe1/1 -> Terminator1/1
  Draw Markers/1 -> Linee Finali/1
  Hough Transform/1 -> Overwrite/1(In)
  Subsystem/1(Punto camera) -> Draw Markers/2
  Linee Laterali/1 -> Linea Centrale/1
  [ILow] -> 2-D FIR Filter/1
  Transpose/1 -> select rho/1, select rho3/1
  Image thresholding/1 -> Hough Transform/1
  Linea Centrale/1 -> Draw Markers/1
  Clip image/1 -> [ILow]
  deg2m/sec/1 -> [REF_DX]  "omega_R"
  Individua linea centrale/1(Linea centrale) -> Subsystem/1(Linea centrale), Linea Centrale/2
  Constant/1 -> convToWheelVel1/1(v(cm/s))
  Selector theta/1 -> [theta]
  2-D FIR Filter/1 -> Image thresholding/1
  PID Controller/1 -> PID_action/1, convToWheelVel1/2(w(deg/s))
  Overwrite/1(Out) -> Find Local Maxima/1
  [rho] -> Hough Lines1/2
  [theta] -> Hough Lines1/1
  Zero-Order Hold3/1 -> Selector rho/1
  Edge Detection1/1 -> Hough Lines1/3
  Selector rho/1 -> [rho]
  [ILow] -> Edge Detection1/1
  Find Local Maxima/1 -> Selector1/1
  deg2m/s/1 -> [REF_SX]  "omega_L"
  [ILow] -> Linee Laterali/1
  Hough Lines1/1 -> Individua linea centrale/1(Matrice punti), Linee Laterali/2
  Hough Transform/3 -> Zero-Order Hold3/1
  convToWheelVel1/2(wr (deg/s)) -> deg2m/sec/1
  Subscribe1/2 -> Read Image1/1
  convToWheelVel1/1(wl (deg/s)) -> deg2m/s/1
  Selector1/1 -> Transpose/1
  Zero-Order Hold2/1 -> Selector theta/1
  Subsystem/2(Distanza) -> [Distanza]
  Hough Transform/2 -> Zero-Order Hold2/1
  select rho3/1 -> Selector theta/2
  select rho/1 -> Selector rho/2
  Scala di grigi/1 -> Clip image/1
  Read Image1/1 -> [RGB], Scala di grigi/1
  [Distanza] -> PID Controller/1
  Manual Switch3/1 -> Bus Assignment/2
  Manual Switch2/1 -> Bus Assignment/3
  [v_s] -> Scope10/1  "v_s"
  [v_r] -> Scope10/2  "v_r"
  [pid_s] -> Scope10/3  "pid_s"
  [pid_r] -> Scope10/4  "pid_r"
  [REF_SX] -> Scope10/5  "ref_s"
  [REF_DX] -> Scope10/6  "ref_d"
  From10/1 -> Sum4/1
  From4/1 -> Data Type Conversion/1
  Data Type Conversion1/1 -> Manual Switch4/2
  Data Type Conversion/1 -> Manual Switch5/1
  From1/1 -> Data Type Conversion1/1
  [u_r] -> Manual Switch2/2
  [u_s] -> Manual Switch3/1
  From2/1 -> Sum2/1
  Constant6/1 -> Manual Switch4/1, Manual Switch5/2
  Bus Assignment1/1 -> Publish1/1
  Manual Switch4/1 -> Bus Assignment1/3
  Blank Message1/1 -> Bus Assignment1/1
  Manual Switch5/1 -> Bus Assignment1/2
  Constant8/1 -> MATLAB Function2/4(thresh_in)
  MATLAB Function1/2(G) -> MATLAB Function2/2(g_in)
  MATLAB Function2/6(riconosciuto) -> Display1/1, [RED_DETECTED]
  MATLAB Function2/3(b_out) -> To Video Display1/3
  MATLAB Function1/3(B) -> MATLAB Function2/3(b_in)
  MATLAB Function2/2(g_out) -> To Video Display1/2
  MATLAB Function2/1(r_out) -> To Video Display1/1
  MATLAB Function1/1(R) -> MATLAB Function2/1(r_in)
  Switch 3/1 -> [azione_r]
  [STOP] -> Switch 6/3, Switch 6/2
  [RED_DETECTED] -> Switch 3/2
  Constant10/1 -> Switch 3/1
  Switch 5/1 -> [u_r]
  [azione_s] -> Switch 6/1
  Constant9/1 -> [STOP]
  [azione_r] -> Switch 5/1
  [STOP] -> Switch 5/3, Switch 5/2
  Switch 6/1 -> [u_s]
  [REF_DX] -> Switch 3/3
  [RGB] -> MATLAB Function1/1(camera)
  [REF_SX] -> Switch 4/3
  [RED_DETECTED] -> Switch 4/2
  Constant11/1 -> Switch 4/1
  Switch 4/1 -> [azione_s]

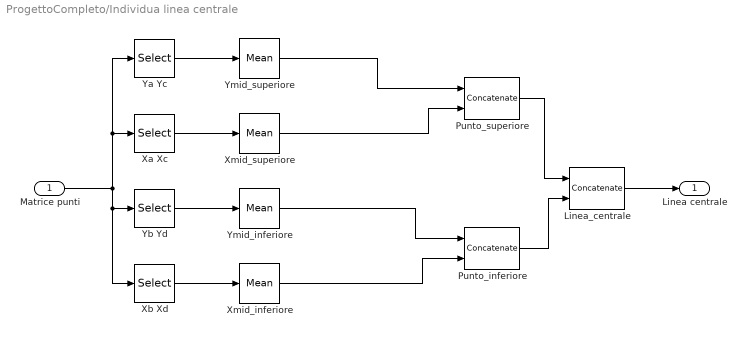
== system ProgettoCompleto/Individua linea centrale ==
  Matrice punti : Inport
  Linea_centrale : Concatenate  Mode=Multidimensional array
  Punto_inferiore : Concatenate  Mode=Multidimensional array
  Punto_superiore : Concatenate  Mode=Multidimensional array
  Xa Xc : Selector  NumberOfDimensions=2  InputPortWidth=3  IndexOptions=Index vector (dialog),Index vector (dialog)  Indices=[1 2],[2]  OutputSizes=1,1
  Xb Xd : Selector  NumberOfDimensions=2  InputPortWidth=3  IndexOptions=Index vector (dialog),Index vector (dialog)  Indices=[1 2],[4]  OutputSizes=1,1
  Xmid_inferiore : dspstat3/Mean  run=off  InputProcessing=Columns as channels (frame based)  reset_popup=None  directionMode=Each column  dimension=1  roiEnable=off  roiType=Rectangles  roiPortion=Entire ROI  roiOutput=Individual statistics for each ROI  roiFlag=off  roundingMode=Floor  overflowMode=off  outputDataTypeStr=Inherit: Same as accumulator  outputMin=[]  outputMax=[]  outputLastDataTypeStr=Inherit: Same as accumulator
  Xmid_superiore : dspstat3/Mean  run=off  InputProcessing=Columns as channels (frame based)  reset_popup=None  directionMode=Each column  dimension=1  roiEnable=off  roiType=Rectangles  roiPortion=Entire ROI  roiOutput=Individual statistics for each ROI  roiFlag=off  roundingMode=Floor  overflowMode=off  outputDataTypeStr=Inherit: Same as accumulator  outputMin=[]  outputMax=[]  outputLastDataTypeStr=Inherit: Same as accumulator
  Ya Yc : Selector  NumberOfDimensions=2  InputPortWidth=3  IndexOptions=Index vector (dialog),Index vector (dialog)  Indices=[1 2],[1]  OutputSizes=1,1
  Yb Yd : Selector  NumberOfDimensions=2  InputPortWidth=3  IndexOptions=Index vector (dialog),Index vector (dialog)  Indices=[1 2],[3]  OutputSizes=1,1
  Ymid_inferiore : dspstat3/Mean  run=off  InputProcessing=Columns as channels (frame based)  reset_popup=None  directionMode=Each column  dimension=1  roiEnable=off  roiType=Rectangles  roiPortion=Entire ROI  roiOutput=Individual statistics for each ROI  roiFlag=off  roundingMode=Floor  overflowMode=off  outputDataTypeStr=Inherit: Same as accumulator  outputMin=[]  outputMax=[]  outputLastDataTypeStr=Inherit: Same as accumulator
  Ymid_superiore : dspstat3/Mean  run=off  InputProcessing=Columns as channels (frame based)  reset_popup=None  directionMode=Each column  dimension=1  roiEnable=off  roiType=Rectangles  roiPortion=Entire ROI  roiOutput=Individual statistics for each ROI  roiFlag=off  roundingMode=Floor  overflowMode=off  outputDataTypeStr=Inherit: Same as accumulator  outputMin=[]  outputMax=[]  outputLastDataTypeStr=Inherit: Same as accumulator
  Linea centrale : Outport
  wires:
  Punto_superiore/1 -> Linea_centrale/1
  Ymid_inferiore/1 -> Punto_inferiore/1
  Ya Yc/1 -> Ymid_superiore/1
  Ymid_superiore/1 -> Punto_superiore/1
  Punto_inferiore/1 -> Linea_centrale/2
  Matrice punti/1 -> Xb Xd/1, Yb Yd/1, Xa Xc/1, Ya Yc/1
  Linea_centrale/1 -> Linea centrale/1
  Yb Yd/1 -> Ymid_inferiore/1
  Xmid_superiore/1 -> Punto_superiore/2
  Xmid_inferiore/1 -> Punto_inferiore/2
  Xb Xd/1 -> Xmid_inferiore/1
  Xa Xc/1 -> Xmid_superiore/1

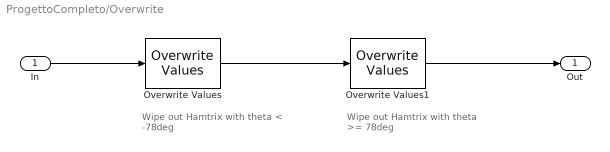
== system ProgettoCompleto/Overwrite ==
  note: Wipe out Hamtrix with
      | theta >=  78deg
  note: Wipe out Hamtrix with
      | theta <  -78deg
  In : Inport
  Overwrite Values : dspmtrx3/Overwrite Values  OverWriteDiag=Submatrix  valFrom2ndIP=Specify via dialog  ConstValue=0  RowSpan=All rows  RowStartMode=First  RowStartIndex=1  RowEndMode=Last  RowEndIndex=1  ColSpan=Range of columns  ColStartMode=First  ColStartIndex=1  ColEndMode=Index  ColEndIndex=12  DiagSpan=Range of elements  DiagStartMode=Index  DiagStartIndex=2  DiagEndMode=Index  DiagEndIndex=4
  Overwrite Values1 : dspmtrx3/Overwrite Values  OverWriteDiag=Submatrix  valFrom2ndIP=Specify via dialog  ConstValue=0  RowSpan=All rows  RowStartMode=First  RowStartIndex=1  RowEndMode=Last  RowEndIndex=1  ColSpan=Range of columns  ColStartMode=Offset from last  ColStartIndex=12  ColEndMode=Last  ColEndIndex=15  DiagSpan=Range of elements  DiagStartMode=Index  DiagStartIndex=2  DiagEndMode=Index  DiagEndIndex=4
  Out : Outport
  wires:
  Overwrite Values/1 -> Overwrite Values1/1
  In/1 -> Overwrite Values/1
  Overwrite Values1/1 -> Out/1

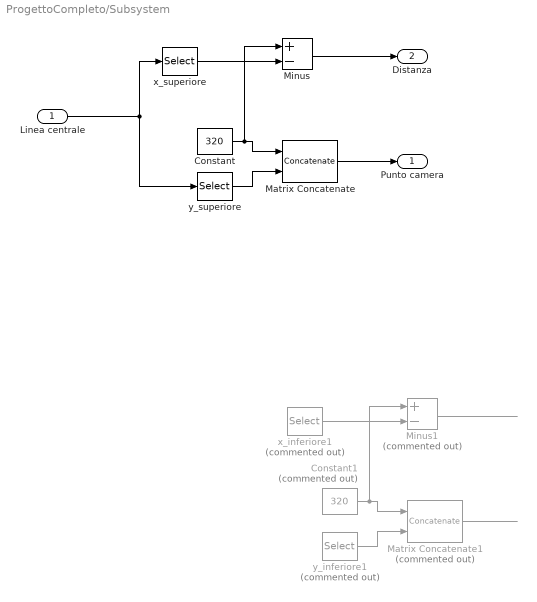
== system ProgettoCompleto/Subsystem ==
  Linea centrale : Inport
  Constant : Constant  Value=320  OutDataTypeStr=int32
  Constant1 : Constant  Commented=on  Value=320  OutDataTypeStr=int32
  Matrix Concatenate : Concatenate  Mode=Multidimensional array
  Matrix Concatenate1 : Concatenate  Commented=on  Mode=Multidimensional array
  Minus : Sum  Inputs=+-
  Minus1 : Sum  Commented=on  Inputs=+-
  x_inferiore1 : Selector  Commented=on  InputPortWidth=4  IndexOptions=Index vector (dialog)  Indices=[3]  OutputSizes=1
  x_superiore : Selector  InputPortWidth=4  IndexOptions=Index vector (dialog)  Indices=[1]  OutputSizes=1
  y_inferiore1 : Selector  Commented=on  InputPortWidth=4  IndexOptions=Index vector (dialog)  Indices=[4]  OutputSizes=1
  y_superiore : Selector  InputPortWidth=4  IndexOptions=Index vector (dialog)  Indices=[2]  OutputSizes=1
  Punto camera : Outport
  Distanza : Outport  Port=2
  wires:
  Minus/1 -> Distanza/1
  Constant/1 -> Minus/1, Matrix Concatenate/1
  Linea centrale/1 -> x_superiore/1, y_superiore/1
  Matrix Concatenate/1 -> Punto camera/1
  y_superiore/1 -> Matrix Concatenate/2
  x_superiore/1 -> Minus/2
  Matrix Concatenate1/1 -> ?
  y_inferiore1/1 -> Matrix Concatenate1/2
  ? -> x_inferiore1/1, y_inferiore1/1
  x_inferiore1/1 -> Minus1/2
  Minus1/1 -> ?
  Constant1/1 -> Minus1/1, Matrix Concatenate1/1

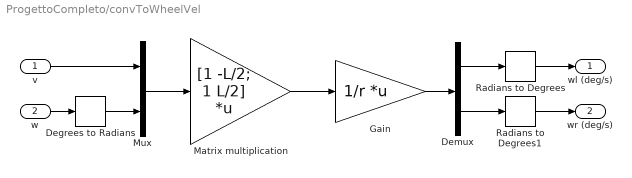
== system ProgettoCompleto/convToWheelVel ==
  v : Inport
  w : Inport  Port=2
  " Gain" : Gain  Gain=1/r  Multiplication=Matrix(K*u)
  Degrees to Radians : simulink_extras/Transformations/Degrees to Radians
  Demux : Demux  Outputs=2
  Matrix multiplication : Gain  Gain=[1 -L/2; 1 L/2]  Multiplication=Matrix(K*u)
  Mux : Mux  Inputs=2
  Radians to Degrees : simulink_extras/Transformations/Radians to Degrees
  Radians to Degrees1 : simulink_extras/Transformations/Radians to Degrees
  wl (deg/s) : Outport  VectorParamsAs1DForOutWhenUnconnected=off
  wr (deg/s) : Outport  Port=2  VectorParamsAs1DForOutWhenUnconnected=off
  wires:
  " Gain"/1 -> Demux/1
  Matrix multiplication/1 -> " Gain"/1
  v/1 -> Mux/1
  Mux/1 -> Matrix multiplication/1
  Demux/1 -> Radians to Degrees/1
  Demux/2 -> Radians to Degrees1/1
  w/1 -> Degrees to Radians/1
  Radians to Degrees/1 -> wl (deg/s)/1
  Radians to Degrees1/1 -> wr (deg/s)/1
  Degrees to Radians/1 -> Mux/2

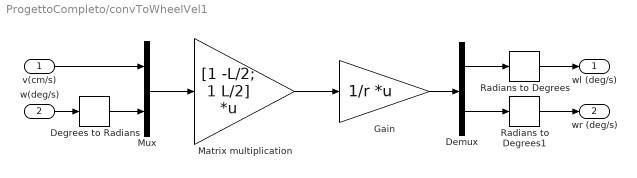
== system ProgettoCompleto/convToWheelVel1 ==
  v(cm/s) : Inport
  w(deg/s) : Inport  Port=2
  " Gain" : Gain  Gain=1/r  Multiplication=Matrix(K*u)
  Degrees to Radians : simulink_extras/Transformations/Degrees to Radians
  Demux : Demux  Outputs=2
  Matrix multiplication : Gain  Gain=[1 -L/2; 1 L/2]  Multiplication=Matrix(K*u)
  Mux : Mux  Inputs=2
  Radians to Degrees : simulink_extras/Transformations/Radians to Degrees
  Radians to Degrees1 : simulink_extras/Transformations/Radians to Degrees
  wl (deg/s) : Outport  VectorParamsAs1DForOutWhenUnconnected=off
  wr (deg/s) : Outport  Port=2  VectorParamsAs1DForOutWhenUnconnected=off
  wires:
  " Gain"/1 -> Demux/1
  Matrix multiplication/1 -> " Gain"/1
  v(cm/s)/1 -> Mux/1
  Mux/1 -> Matrix multiplication/1
  Demux/1 -> Radians to Degrees/1
  Demux/2 -> Radians to Degrees1/1
  w(deg/s)/1 -> Degrees to Radians/1
  Radians to Degrees/1 -> wl (deg/s)/1
  Radians to Degrees1/1 -> wr (deg/s)/1
  Degrees to Radians/1 -> Mux/2

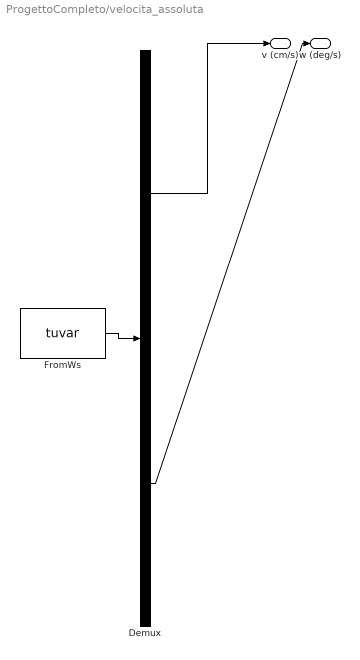
== system ProgettoCompleto/velocita_assoluta ==
  Demux : Demux  Tag=STV Demux  Outputs=2
      settings: DisplayOption=none
  FromWs : FromWorkspace  Tag=STV FromWs  VariableName=tuvar
      SigBuilderData=|
      | common.afterFinalStr = 'Extrapolate'
      | common.sampleTime = 0
      | dataSet.timeRange = [0 200]
      | dataSet.name = 'Group 1'
      | sbobj.Groups.Name = 'Group 1'
      | sbobj.Groups.Signals(1).Name = 'v (cm/s)'
      | sbobj.Groups.Signals(1).XData = [0 51.2 51.2 89 89 200]
      | sbobj.Groups.Signals(1).YData = [0 0 10 10 0 0]
      | sbobj.Groups.Signals(2).Name = 'w (deg/s)'
      | sbobj.Groups.Signals(2).XData = [0 20 21 24 24.4 200]
      | sbobj.Groups.Signals(2).YData = [0 0 0 0 0 0]
      | sbobj.Groups.TimeRange = [0 200]
  v (cm/s) : Outport  Tag=STV Outport
  w (deg/s) : Outport  Tag=STV Outport  Port=2
  wires:
  FromWs/1 -> Demux/1
  Demux/1 -> v (cm/s)/1
  Demux/2 -> w (deg/s)/1

== matlab function ProgettoCompleto/MATLAB Function1 ==
  data: camera input; R output; G output; B output
function [R,G,B] = fcn(camera)


[R,G,B]=imsplit(camera);

== matlab function ProgettoCompleto/MATLAB Function2 ==
  data: r_in input; r_out output; g_in input; b_in input; thresh_in input; g_out output; b_out output; xm output; ym output; riconosciuto output
function [r_out, g_out, b_out, xm, ym, riconosciuto] = fcn(r_in, g_in, b_in, thresh_in)
    % Get RGB color
    r = r_in;
    g = g_in;
    b = b_in;
    thresh = thresh_in;
    % Calcola il canale rosso modificato
    justRed = r - g/2 - b/2;
    % Soglia dell'immagine
    bw = justRed > thresh;
    % Applica una condizione aggiuntiva basata sui valori dei canali RGB
    redCondition = (r > 120) & (g < 100) & (b < 100);
    bw = bw & redCondition;
    % Trova il centro
    [x, y] = find(bw);
    xm = mean(x);
    ym = mean(y);
    % Crea il rettangolo verde
    xx = max(1, xm - 5):min(xm + 5, size(bw, 1));
    yy = max(1, ym - 5):min(ym + 5, size(bw, 2));
    bwbw = zeros(size(bw), 'uint8');
    bwbw(uint16(xx), uint16(yy)) = 255;
    % Sovrapposizione dei rettangoli all'immagine originale
    r_out = uint8(double(r_in) - double(bwbw));
    g_out = uint8(double(g_in) + double(bwbw));
    b_out = uint8(double(b_in) - double(bwbw));
    % Verifica se il rosso è stato riconosciuto
    if any(bw(:))
        riconosciuto = 1;
    else
        riconosciuto = 0;
    end
end

== stateflow chart ProgettoCompleto/Chart ==
  state GoRight
    entry: v = 2
    w = -8
  state GoLeft
    entry: v = 2
    w = 8
  state StraightOn
    entry: v = 8
    w = 0
  StraightOn -> GoRight [order 2] : [distanza < -eps]
  GoRight -> StraightOn : [distanza >= -eps]
  StraightOn -> GoLeft [order 1] : [distanza > eps]
  GoLeft -> StraightOn : [distanza <= eps]
  (default) -> StraightOn
  data: distanza input; v output; w output; eps constant double =5
